simulink model "FunctionCall_Subsystem"  (R2024a)
settings: Solver=FixedStepDiscrete  StartTime=0.0  StopTime=10.0  RelTol=1e-3
libraries: simulink x3
settings Model: Creator=VICTUS  LastModifiedBy=VICTUS
settings OptimizationCC: DefaultParameterBehavior=Inlined  UseDivisionForNetSlopeComputation=on  GainParamInheritBuiltInType=on  UseFloatMulNetSlope=on  InlineInvariantSignals=on  PassReuseOutputArgsAs=Individual arguments  ZeroExternalMemoryAtStartup=off  ZeroInternalMemoryAtStartup=off  NoFixptDivByZeroProtection=on  EfficientFloat2IntCast=on  LifeSpan=1  OptimizeBlockOrder=speed  DifferentSizesBufferReuse=on  EfficientTunableParamExpr=on
settings DebuggingCC: ParameterTunabilityLossMsg=error
settings HardwareCC: ProdBitPerPointer=32  ProdBitPerSizeT=32  ProdBitPerPtrDiffT=32  ProdLargestAtomicInteger=Long  ProdWordSize=32  ProdLongLongMode=on  ProdHWDeviceType=ARM Compatible->ARM 10
settings SFSimCC: MATLABDynamicMemAlloc=off
settings RTWCC: Description=Embedded Coder  SystemTargetFile=ert.tlc  TemplateMakefile=ert_default_tmf
settings CodeAppCC: ForceParamTrailComments=on  IgnoreCustomStorageClasses=off  OperatorAnnotations=on  SimulinkDataObjDesc=on  SFDataObjDesc=on  CustomSymbolStrGlobalVar=rt$N$M  CustomSymbolStrType=$N$M  CustomSymbolStrFcn=$N$M$F  CustomSymbolStrMacro=$N$M  InsertBlockDesc=on
settings ERTTargetCC: TargetLangStandard=C99 (ISO)  GenerateSampleERTMain=on  IncludeMdlTerminateFcn=off  CombineSignalStateStructs=on  SupportAbsoluteTime=off  SupportComplex=off  SupportNonInlinedSFcns=on  InlinedParameterPlacement=NonHierarchical  ERTCustomFileTemplate=example_file_process.tlc  ERTFilePackagingFormat=CompactWithDataFile

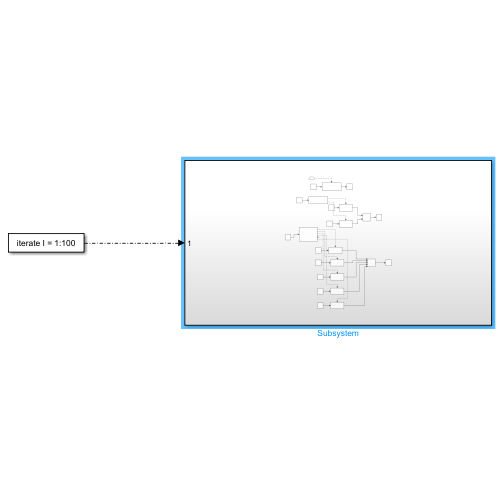
[thumbnail: Simulink's stored preview of the top-level diagram]
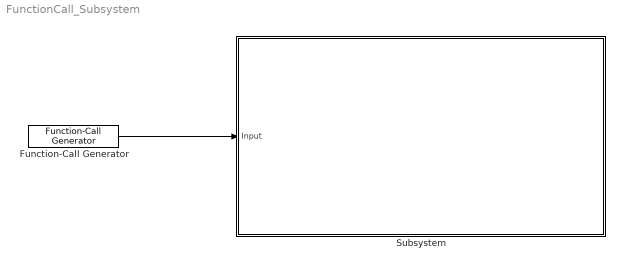
== system FunctionCall_Subsystem ==
  Function-Call Generator : simulink/Ports & Subsystems/Function-Call Generator  sample_time=1  numberOfIterations=100  DisallowWideOutput=off
  Subsystem : Subsystem
  wires:
  Function-Call Generator/1 -> Subsystem/1(Input)

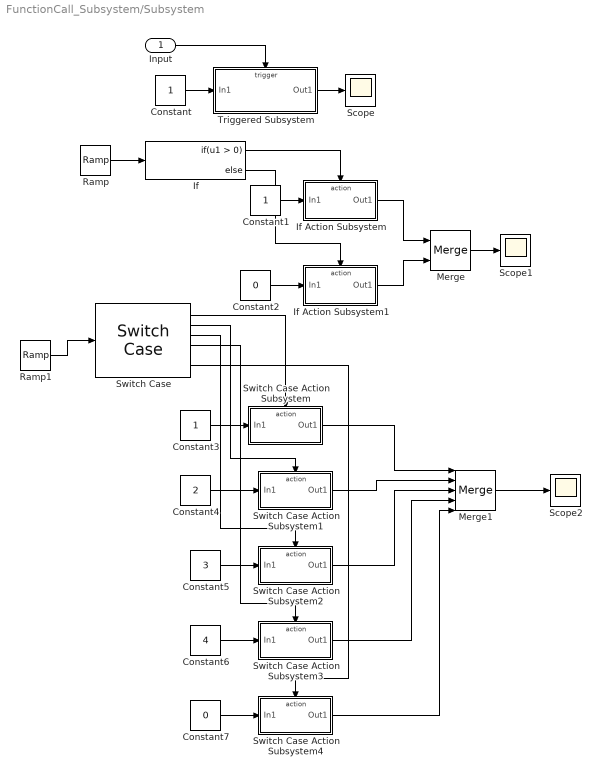
== system FunctionCall_Subsystem/Subsystem ==
  Input : Inport
  Constant : Constant
  Constant1 : Constant
  Constant2 : Constant  Value=0
  Constant3 : Constant
  Constant4 : Constant  Value=2
  Constant5 : Constant  Value=3
  Constant6 : Constant  Value=4
  Constant7 : Constant  Value=0
  If : If
  If Action Subsystem : Subsystem  TreatAsAtomicUnit=on
  If Action Subsystem1 : Subsystem  TreatAsAtomicUnit=on
  Merge : Merge
  Merge1 : Merge  Inputs=5
  Ramp : simulink/Sources/Ramp  slope=1  start=0  InitialOutput=0
  Ramp1 : simulink/Sources/Ramp  slope=1  start=0  InitialOutput=0
  Scope : Scope
  Scope1 : Scope
  Scope2 : Scope
  Switch Case : SwitchCase  CaseConditions={1,2,3,4,5}
  Switch Case Action Subsystem : Subsystem  TreatAsAtomicUnit=on
  Switch Case Action Subsystem1 : Subsystem  TreatAsAtomicUnit=on
  Switch Case Action Subsystem2 : Subsystem  TreatAsAtomicUnit=on
  Switch Case Action Subsystem3 : Subsystem  TreatAsAtomicUnit=on
  Switch Case Action Subsystem4 : Subsystem  TreatAsAtomicUnit=on
  Triggered Subsystem : Subsystem  TreatAsAtomicUnit=on
  wires:
  Input/1 -> Triggered Subsystem/Trigger
  Triggered Subsystem/1(Out1) -> Scope/1
  Constant/1 -> Triggered Subsystem/1(In1)
  If/1 -> If Action Subsystem/Action
  Ramp/1 -> If/1
  If/2 -> If Action Subsystem1/Action
  Constant1/1 -> If Action Subsystem/1(In1)
  Constant2/1 -> If Action Subsystem1/1(In1)
  If Action Subsystem/1(Out1) -> Merge/1
  If Action Subsystem1/1(Out1) -> Merge/2
  Merge/1 -> Scope1/1
  Switch Case/1 -> Switch Case Action Subsystem/Action
  Ramp1/1 -> Switch Case/1
  Constant3/1 -> Switch Case Action Subsystem/1(In1)
  Switch Case/2 -> Switch Case Action Subsystem1/Action
  Constant4/1 -> Switch Case Action Subsystem1/1(In1)
  Switch Case/3 -> Switch Case Action Subsystem2/Action
  Constant5/1 -> Switch Case Action Subsystem2/1(In1)
  Constant6/1 -> Switch Case Action Subsystem3/1(In1)
  Switch Case/4 -> Switch Case Action Subsystem3/Action
  Switch Case Action Subsystem/1(Out1) -> Merge1/1
  Switch Case Action Subsystem1/1(Out1) -> Merge1/2
  Switch Case Action Subsystem2/1(Out1) -> Merge1/3
  Switch Case Action Subsystem3/1(Out1) -> Merge1/4
  Merge1/1 -> Scope2/1
  Switch Case/6 -> Switch Case Action Subsystem4/Action
  Switch Case Action Subsystem4/1(Out1) -> Merge1/5
  Constant7/1 -> Switch Case Action Subsystem4/1(In1)

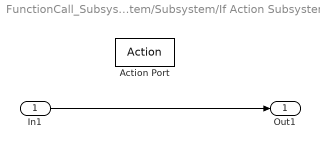
== system FunctionCall_Subsystem/Subsystem/If Action Subsystem ==
  In1 : Inport
  Action Port : ActionPort  ActionPortLabel=if(u1 > 0)
  Out1 : Outport
  wires:
  In1/1 -> Out1/1

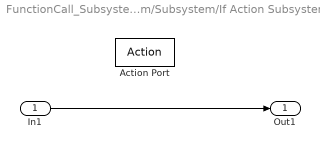
== system FunctionCall_Subsystem/Subsystem/If Action Subsystem1 ==
  In1 : Inport
  Action Port : ActionPort  ActionPortLabel=else
  Out1 : Outport
  wires:
  In1/1 -> Out1/1

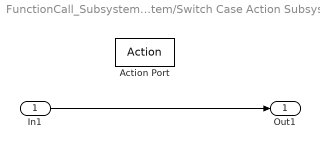
== system FunctionCall_Subsystem/Subsystem/Switch Case Action Subsystem ==
  In1 : Inport
  Action Port : ActionPort  ActionPortLabel=case [ 1 ]:
  Out1 : Outport
  wires:
  In1/1 -> Out1/1

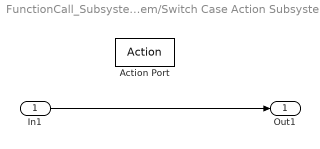
== system FunctionCall_Subsystem/Subsystem/Switch Case Action Subsystem1 ==
  In1 : Inport
  Action Port : ActionPort  ActionPortLabel=case [ 2 ]:
  Out1 : Outport
  wires:
  In1/1 -> Out1/1

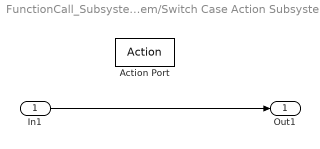
== system FunctionCall_Subsystem/Subsystem/Switch Case Action Subsystem2 ==
  In1 : Inport
  Action Port : ActionPort  ActionPortLabel=case [ 3 ]:
  Out1 : Outport
  wires:
  In1/1 -> Out1/1

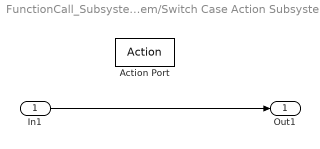
== system FunctionCall_Subsystem/Subsystem/Switch Case Action Subsystem3 ==
  In1 : Inport
  Action Port : ActionPort  ActionPortLabel=case [ 4 ]:
  Out1 : Outport
  wires:
  In1/1 -> Out1/1

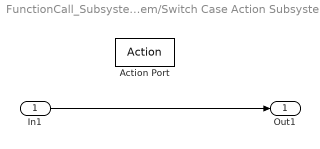
== system FunctionCall_Subsystem/Subsystem/Switch Case Action Subsystem4 ==
  In1 : Inport
  Action Port : ActionPort  ActionPortLabel=default:
  Out1 : Outport
  wires:
  In1/1 -> Out1/1

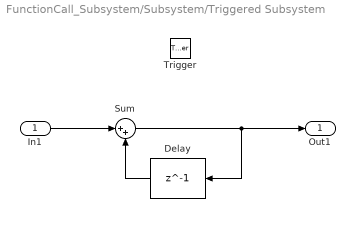
== system FunctionCall_Subsystem/Subsystem/Triggered Subsystem ==
  In1 : Inport
  Trigger : TriggerPort  TriggerType=function-call  VariantControl=(inherit)
  Delay : Delay  DelayLength=1  InitialCondition=0  UseCircularBuffer=on
  Sum : Sum  Inputs=|++
  Out1 : Outport
  wires:
  Sum/1 -> Delay/1, Out1/1
  In1/1 -> Sum/1
  Delay/1 -> Sum/2
